simulink model "example11_1"  (R2022b)
settings: Solver=FixedStepAuto  StartTime=0.0  StopTime=10.0  FixedStep=0.01  RelTol=1e-3
InitFcn:
  | example11_1_params;
values from neighbouring files (symbols this model uses):
  A = [0 1 ; 20.6 0]    [example11_1_params.m]
  B = [0 ; 1]    [example11_1_params.m]
  C = [1 1]    [example11_1_params.m]
  G = acker(A',C',[-8; -8])'    [example11_1_params.m]
  K = place(A,B,[-1.8+2.4i; -1.8-2.4i])    [example11_1_params.m]
  x0 = [0.1 ; 0]    [example11_1_params.m]
  x0hat = [0 ; 0]    [example11_1_params.m]
settings Model: Creator=vcichella  LastModifiedBy=vcichella

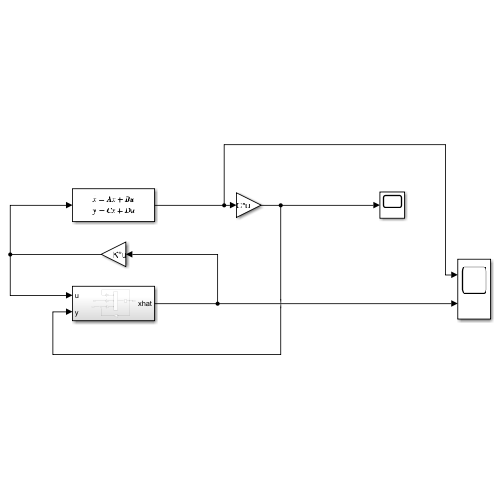
[thumbnail: Simulink's stored preview of the top-level diagram]
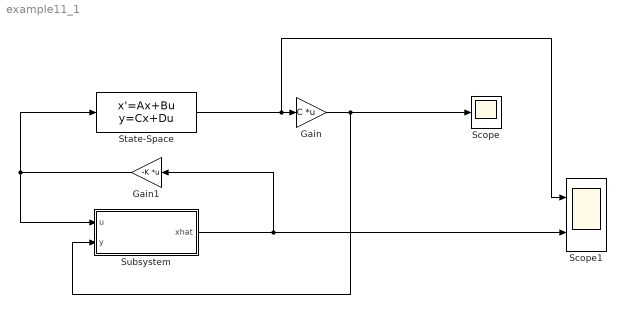
== system example11_1 ==
  Gain : Gain  Gain=C  Multiplication=Matrix(K*u)
  Gain1 : Gain  Gain=-K  Multiplication=Matrix(K*u)
  Scope : Scope
  Scope1 : Scope  NumInputPorts=2
  State-Space : StateSpace  A=A  B=B  C=eye(2)  D=zeros(2,1)  InitialCondition=x0
  Subsystem : Subsystem
  wires:
  State-Space/1 -> Scope1/1, Gain/1
  Gain/1 -> Scope/1, Subsystem/2(y)
  Subsystem/1(xhat) -> Gain1/1, Scope1/2
  Gain1/1 -> Subsystem/1(u), State-Space/1

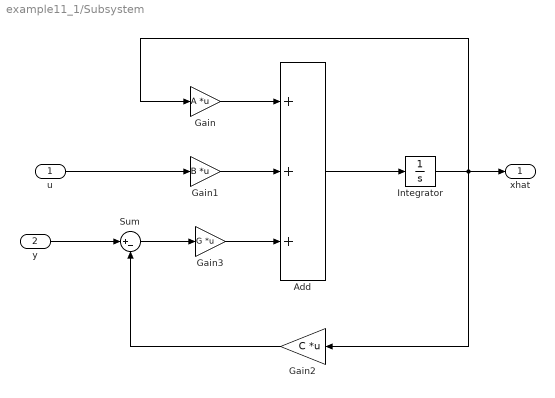
== system example11_1/Subsystem ==
  u : Inport
  y : Inport  Port=2
  Add : Sum  Inputs=+++
  Gain : Gain  Gain=A  Multiplication=Matrix(K*u)
  Gain1 : Gain  Gain=B  Multiplication=Matrix(K*u)
  Gain2 : Gain  Gain=C  Multiplication=Matrix(K*u)
  Gain3 : Gain  Gain=G  Multiplication=Matrix(K*u)
  Integrator : Integrator  InitialCondition=x0hat
  Sum : Sum  Inputs=|+-
  xhat : Outport
  wires:
  Integrator/1 -> Gain2/1, Gain/1, xhat/1
  Add/1 -> Integrator/1
  Gain/1 -> Add/1
  Gain1/1 -> Add/2
  u/1 -> Gain1/1
  y/1 -> Sum/1
  Gain2/1 -> Sum/2
  Sum/1 -> Gain3/1
  Gain3/1 -> Add/3
